simulink library "dspsrcs4"  (Simulink 6.0)
settings: Solver=ode45  SolverMode=SingleTasking  StartTime=0.0  StopTime=10.0  RelTol=1e-3
undefined symbols (not defined in the file or in its folder): dTypeID, Low
libraries: dspsigattribs x3, dspmtrx3 x2, dspswit3 x1
settings Model: RequirementInfo=9  CovMetricSettings=d  Creator=lelas  LastModifiedBy=sconahan  ExtModeAutoUpdateStatusClock=off
settings DataIOCC: SignalLoggingName=logsOut
settings OptimizationCC: BooleanDataType=off
settings DebuggingCC: CheckExecutionContextPreStartOutputMsg=on  CheckExecutionContextRuntimeOutputMsg=on  SolverPrmCheckMsg=none
settings HardwareCC: TargetUnknown=on
settings ModelReferenceCC: UpdateModelReferenceTargets=IfOutOfDate
settings SFSimCC: SFSimApplyToAllLibs=on  SFSimBuildMode=Incremental

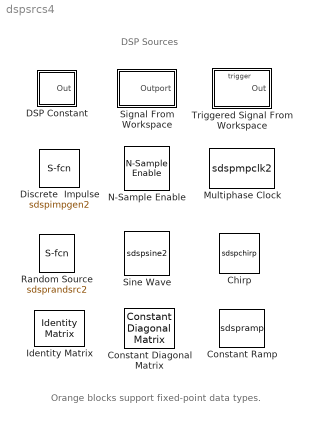
== system dspsrcs4 ==
  note: DSP Sources
  note: Orange blocks support fixed-point data types.
  Chirp : S-Function  FunctionName=sdspchirp  Parameters=sweep, mode, f0, f1, t1, Tsweep, phase, Ts, spf, beta, fmin,datatype  mask(Chirp){sweep=Linear, mode=Unidirectional, f0=1000, f1=4000, t1=1, Tsweep=1, phase=0, Ts=1/8000, spf=1, datatype=Double}
      mask prompts: sweep "Frequency sweep:"; mode "Sweep mode:"; f0 "Initial frequency (Hz):"; f1 "Target frequency (Hz):"; t1 "Target time (sec):"; Tsweep "Sweep time (sec):"; phase "Initial phase (radians):"; Ts "Sample time:"; spf "Samples per frame:"; datatype "Output data type:"
      mask help: Linear, Logarithmic, and Quadratic modes generate a swept-frequency cosine with instantaneous frequency values specified by the frequency and time parameters. The Swept cosine mode generates a swept-frequency cosine with a linear instantaneous output frequency that may differ from the one specified by the frequency and time parameters.
      mask init:
      | [t,y,txt] = dspblkchirp2('icon');
      | [beta,fmin] = dspblkchirp2('param',sweep, f0, f1, t1,Tsweep);
      mask Help: web(dspbhelp);
      mask StyleString: popup(Swept cosine|Linear|Logarithmic|Quadratic),popup(Unidirectional|Bidirectional),edit,edit,edit,edit,edit,edit,edit,popup(Double|Single)
      mask Display:
      | plot(t,y);
      | text(.2,.85,txt)
  Constant Diagonal Matrix : dspmtrx3/Constant Diagonal Matrix  q=ones(1,3)  frame=off  dataType=Inherit from 'Constant(s) along diagonal'  isSigned=on  wordLen=16  udDataType=sfix(16)  fracBitsMode=Best precision  numFracBits=15
  Constant Ramp : S-Function  FunctionName=sdspramp  Parameters=L, Slope, Offset,isCustomFloat,isSigned,dTypeID,wordLength,fracBits,fracBitsMode  mask(Constant Ramp){L=Rows, Slope=1, Offset=0, additionalParams=off, allowOverrides=on, dataType=Same as input, isSigned=on, wordLen=16, udDataType=sfix(16), fracBitsMode=Best precision, numFracBits=15}
      mask prompts: L "Ramp length equals number of:"; additionalParams "------- Show additional parameters --------"; allowOverrides "Allow overrides from DSP Fixed-Point Attributes blocks"; dataType "Output data type:"; isSigned "Signed"; wordLen "Word length:"; udDataType "User-defined data type (e.g. sfix(16), float('single')):"; fracBitsMode "Set fraction length in output to:"; numFracBits "Fraction length:"
      mask help:
      | Generate a ramp of length L, where L is either the number of rows or the number of columns of the input to the block.  Specify whether L is equal to the number of input rows or columns using the 'Ramp length equals number of' parameter.
      |
      | The output of this block is calculated using
      | output = [0:L-1] * slope + offset
      |
      | Note: Use the Ramp block in the Simulink Sources library to generate a ramp without providing block inputs.
      mask init:
      | x = [.1 .9];
      | if ~isa(Slope,'double')
      | 	s = 1;
      | else
      | 	s = Slope;
      | end
      | if (s >= 0), y =  s * [0 1];
      | else,   y =  s * [-1 0];  end;
      | [dtInfo,dTypeID]=dspblkramp('init');
      | isSigned=dtInfo.DataTypeIsSigned;
      | isCustomFloat=dtInfo.DataTypeIsCustomFloat;
      | wordLength=dtInfo.DataTypeWordLength;
      | fracBits=dtInfo.DataTypeFracOrMantBits;
      settings: CopyFcn=dspfixptcopycallback
      mask Help: web(dspbhelp);
      mask StyleString: popup(Rows|Columns),edit,edit,checkbox,checkbox,popup(Same as input|double|single|int8|uint8|int16|uint16|int32|uint32|boolean|Fixed-point|User-defined|Inherit via back propagation),checkbox,edit,edit,popup(Best precision|User-defined),edit
      mask CallbackString: |||||dspblkramp;|||dspblkramp;|dspblkramp;|
      mask TabNameString: Main,Main,Main,Main,Main,Data Types,Data Types,Data Types,Data Types,Data Types,Data Types
      mask Display: plot(x,y)
  DSP Constant : Subsystem  PropExecContextAcrossSSBoundary=on  mask(DSP Constant){Value=1, SampleMode=Discrete, discreteOutput=Sample-based, continuousOutput=Sample-based, sampTime=1, framePeriod=2, additionalParams=off, allowOverrides=on, dataType=Inherit from 'Constant value', isSigned=on, wordLen=16, udDataType=sfix(16), fracBitsMode=Best precision, numFracBits=15, InterpretAs1D=-inf, Ts=-inf, FramebasedOutput=-inf}
      mask prompts: Value "Constant value:"; SampleMode "Sample mode:"; discreteOutput "Output:"; continuousOutput "Output:"; sampTime "Sample time:"; framePeriod "Frame period:"; additionalParams "------- Show additional parameters --------"; allowOverrides "Allow overrides from DSP Fixed-Point Attributes blocks"; dataType "Output data type:"; isSigned "Signed"; wordLen "Word length:"; udDataType "User-defined data type:"; fracBitsMode "Set fraction length in output to:"; numFracBits "Fraction length:"; InterpretAs1D "old Interpret as 1D checkbox"; Ts "old Sample time/Frame period"; FramebasedOutput "old Frame-based output checkbox"
      mask help: Output a discrete-time or continuous-time constant.
      mask init:
      | dspblkdspconst2('init');
      | dspblkdspconst2('update');
      settings: CopyFcn=dspfixptcopycallback
      mask Help: web(dspbhelp);
      mask StyleString: edit,popup(Discrete|Continuous),popup(Sample-based (interpret vectors as 1-D)|Sample-based|Frame-based),popup(Sample-based (interpret vectors as 1-D)|Sample-based),edit,edit,checkbox,checkbox,popup(double|single|int8|uint8|int16|uint16|int32|uint32|boolean|Fixed-point|User-defined|Inherit from 'Constant value'|Inherit via back propagation),checkbox,edit,edit,popup(Best precision|User-defined),edit,edit,edit,edit
      mask CallbackString: |dspblkdspconst2;|dspblkdspconst2;|dspblkdspconst2;|||||dspblkdspconst2;|||dspblkdspconst2;|dspblkdspconst2;||||
      mask TabNameString: Main,Main,Main,Main,Main,Main,Main,Main,Data Types,Data Types,Data Types,Data Types,Data Types,Data Types,Main,Main,Main
      mask Display: disp(&1);
  Discrete  Impulse : S-Function  FunctionName=sdspimpgen2  Parameters=Delay, SampleTime,FrameSample,isCustomFloat,isSigned,dTypeID,wordLength,fracLength,[0 1]  mask(Discrete Impulse ){Delay=0, SampleTime=1, FrameSample=1, additionalParams=off, allowOverrides=on, dataType=double, isSigned=on, wordLen=16, udDataType=sfix(16), fracBitsMode=Best precision, numFracBits=15}
      mask prompts: Delay "Delay (samples):"; SampleTime "Sample time:"; FrameSample "Samples per frame:"; additionalParams "------- Show additional parameters --------"; allowOverrides "Allow overrides from DSP Fixed-Point Attributes blocks"; dataType "Output data type:"; isSigned "Signed"; wordLen "Word length:"; udDataType "User-defined data type (e.g. sfix(16), float('single')):"; fracBitsMode "Set fraction length in output to:"; numFracBits "Fraction length:"
      mask help: Output a discrete unit impulse. The impulse will be offset by the number of samples in the Delay parameter.
      mask init:
      | [x,y]=dspblkimpgen2('icon');
      | [dtInfo,dTypeID]=dspblkimpgen2('init');
      | isSigned=dtInfo.DataTypeIsSigned;
      | isCustomFloat=dtInfo.DataTypeIsCustomFloat;
      | wordLength=dtInfo.DataTypeWordLength;
      | fracLength=dtInfo.DataTypeFracOrMantBits;
      settings: CopyFcn=dspfixptcopycallback
      mask Help: web(dspbhelp);
      mask StyleString: edit,edit,edit,checkbox,checkbox,popup(double|single|int8|uint8|int16|uint16|int32|uint32|boolean|Fixed-point|User-defined|Inherit via back propagation),checkbox,edit,edit,popup(Best precision|User-defined),edit
      mask CallbackString: |||||dspblkimpgen2|||dspblkimpgen2|dspblkimpgen2|
      mask TabNameString: Main,Main,Main,Main,Main,Data Types,Data Types,Data Types,Data Types,Data Types,Data Types
      mask Display: plot(x,y)
  Identity Matrix : dspmtrx3/Identity Matrix  Inherit=off  N=5  Ts=1  dataType=double  isSigned=on  wordLen=16  udDataType=sfix(16)  fracBitsMode=Best precision  numFracBits=15
  Multiphase Clock : S-Function  FunctionName=sdspmpclk2  Parameters=ClkFreq, NumPhases, ActiveLevel, DutyCycle, StartPhase,DataType  mask(Multiphase Clock){ClkFreq=1, NumPhases=4, StartPhase=1, DutyCycle=3, ActiveLevel=High (1), DataType=Logical}
      mask prompts: ClkFreq "Clock frequency (Hz):"; NumPhases "Number of phases, N:"; StartPhase "Starting phase (1 to N):"; DutyCycle "Number of phase intervals over which clock is active (1 to N-1):"; ActiveLevel "Active level (polarity):"; DataType "Output data type"
      mask help: Generate a vector of N binary signals representing the N clock phases.
      mask init:
      | if isempty(NumPhases), s=&2;
      | else s=num2str(NumPhases);
      | end
      | s=[s '-Phase\nClock'];
      settings: CopyFcn=dspfixptcopycallback
      mask Help: web(dspbhelp);
      mask StyleString: edit,edit,edit,edit,popup(High (1)|Low (0)),popup(Logical|Boolean)
      mask Display: disp(s)
  N-Sample Enable : dspswit3/N-Sample Enable  N=8  ActiveLevel=Low (0)  reset=off  TriggerType=Rising edge  Ts=1  DataType=Logical
  Random Source : S-Function  FunctionName=sdsprandsrc2  Parameters=SrcType,NormMethod,double(CltLength),double(Min),double(Max),Mean,double(Var),RepMode,rawSeed,transformSeed,Inherit,SampMode,double(SampTime),SampFrame,DataType,OutComplex  mask(Random Source){SrcType=Uniform, NormMethod=Ziggurat, CltLength=12, Min=0, Max=1, Mean=0, Var=1, RepMode=Not repeatable, rawSeed=1, Inherit=off, SampMode=Discrete, SampTime=1, SampFrame=1, DataType=Double, OutComplex=Real}
      mask prompts: SrcType "Source type:"; NormMethod "Method:"; CltLength "Number of uniform values to sum:"; Min "Minimum:"; Max "Maximum:"; Var "Variance:"; RepMode "Repeatability:"; rawSeed "Initial seed:"; Inherit "Inherit output port attributes"; SampMode "Sample mode:"; SampTime "Sample time:"; SampFrame "Samples per frame:"; DataType "Output data type:"; OutComplex "Complexity:"
      mask help: Output a random signal with uniform or Gaussian (normal) distribution. Set output repeatability to Nonrepeatable (block randomly selects initial seed every time simulation starts), Repeatable (block randomly selects initial seed once and uses it every time simulation starts), or Specify seed (block uses specified initial seed every time simulation starts, producing repeatable output).
      mask init:
      | [x,y]=dspblkrandsrc2('icon');
      | if RepMode == 1
      | 	transformSeed=[];
      | else
      | 	transformSeed=eval(dspblkrandsrc2('seed'),'rawSeed');
      | end
      mask Help: web(dspbhelp);
      mask StyleString: popup(Uniform|Gaussian),popup(Ziggurat|Sum of uniform values),edit,edit,edit,edit,edit,popup(Specify seed|Repeatable|Not repeatable),edit,checkbox,popup(Discrete|Continuous),edit,edit,popup(Double|Single),popup(Real|Complex)
      mask CallbackString:
      | dspblkrandsrc2;|dspblkrandsrc2;
      | ||||||dspblkrandsrc2;||dspblkrandsrc2;|dspblkrandsrc2;||||
      mask Display: plot(x,y);
  Signal From Workspace : Subsystem  PropExecContextAcrossSSBoundary=on  mask(Signal From Workspace){X=1:10, Ts=1, nsamps=1, OutputAfterFinalValue=Setting to zero}
      mask prompts: X "Signal:"; Ts "Sample time:"; nsamps "Samples per frame:"; OutputAfterFinalValue "Form output after final data value by:"
      mask help:
      | Output signal samples obtained from the MATLAB workspace at successive sample times.  A signal matrix is interpreted as having one channel per column.  Signal columns may be buffered into frames by specifying a number of samples per frame greater than 1.
      |
      | An M x N x P signal array outputs M x N matrices at successive sample times.  The samples per frame must be equal to 1 for 3 dimensional signal arrays.
      mask init:
      | [s,Ts] = dspblksfw2('init', X,Ts,nsamps);
      settings: CopyFcn=dspfixptcopycallback
      mask Help: web(dspbhelp);
      mask StyleString: edit,edit,edit,popup(Setting to zero|Holding final value|Cyclic repetition)
      mask Display: disp(&1)
  Sine Wave : S-Function  FunctionName=sdspsine2  Parameters=Amplitude,Frequency,Phase,SampleMode,OutComplex,CompMethod,SampleTime,SamplesPerFrame,ResetState,TableSize,isCustomFloat,isSigned,dTypeID,wordLength,fracBits  mask(Sine Wave){Amplitude=1, Frequency=100, Phase=0, SampleMode=Discrete, OutComplex=Real, CompMethod=Trigonometric fcn, TableSize=Speed, SampleTime=1/1000, SamplesPerFrame=1, additionalParams=off, allowOverrides=on, dataType=double, wordLen=16, udDataType=sfix(16), fracBitsMode=Best precision, numFracBits=15, ResetState=Restart at time zero}
      mask prompts: Frequency "Frequency (Hz):"; Phase "Phase offset (rad):"; SampleMode "Sample mode:"; OutComplex "Output complexity:"; CompMethod "Computation method:"; TableSize "Optimize table for:"; SampleTime "Sample time:"; SamplesPerFrame "Samples per frame:"; additionalParams "------- Show additional parameters --------"; allowOverrides "Allow overrides from DSP Fixed-Point Attributes blocks"; dataType "Output data type:"; wordLen "Word length:"; udDataType "User-defined data type (e.g. sfix(16), float('single')):"; fracBitsMode "Set fraction length in output to:"; numFracBits "Fraction length:"; ResetState "Resetting states when re-enabled:"
      mask help: Output samples of a sinusoid. To generate more than one sinusoid simultaneously, enter a vector of values for the Amplitude, Frequency, and Phase offset parameters.
      mask init:
      | [x,y] = dspblksine('icon');
      | [dtInfo,dTypeID]=dspblksine('init');
      | isSigned=dtInfo.DataTypeIsSigned;
      | isCustomFloat=dtInfo.DataTypeIsCustomFloat;
      | wordLength=dtInfo.DataTypeWordLength;
      | fracBits=dtInfo.DataTypeFracOrMantBits;
      | dType=dataType;
      settings: CopyFcn=dspfixptcopycallback
      mask Help: web(dspbhelp);
      mask StyleString: edit,edit,edit,popup(Discrete|Continuous),popup(Real|Complex),popup(Trigonometric fcn|Table lookup|Differential),popup(Speed|Memory),edit,edit,checkbox,checkbox,popup(double|single|Fixed-point|User-defined|Inherit via back propagation),edit,edit,popup(Best precision|User-defined),edit,popup(Restart at time zero|Catch up to simulation time)
      mask CallbackString: |||dspblksine;||dspblksine;||||||dspblksine||dspblksine|dspblksine||
      mask TabNameString: Main,Main,Main,Main,Main,Main,Main,Main,Main,Main,Main,Data Types,Data Types,Data Types,Data Types,Data Types,Main
      mask Display:
      | plot(x,y)
      | text(3.25,.75,'DSP');
  Triggered Signal From Workspace : Subsystem  TreatAsAtomicUnit=on  PropExecContextAcrossSSBoundary=on  mask(Triggered Signal From Workspace){Signal=1:10, TriggerType=Falling edge, ic=0, SamplesPerFrame=1, OutputAfterFinalValue=Setting to zero}
      mask prompts: TriggerType "Trigger type:"; ic "Initial output:"; SamplesPerFrame "Samples per frame:"; OutputAfterFinalValue "Form output after final data value by:"
      mask help: Output successive signal samples obtained from the MATLAB workspace when a trigger event occurs. A signal matrix is interpreted as having one channel per column. Signal columns may be buffered into frames by specifying a number of samples per frame greater than 1. An M x N x P signal array outputs M x N matrices when a trigger event occurs. The samples per frame must be equal to 1 for 3 dimensional signal arrays.
      mask init:
      | s = dspblktsfw2('init', Signal,SamplesPerFrame);
      settings: CopyFcn=dspfixptcopycallback
      mask Help: web(dspbhelp);
      mask StyleString: edit,popup(Rising edge|Falling edge|Either edge),edit,edit,popup(Setting to zero|Holding final value|Cyclic repetition)
      mask Display: disp(&1);

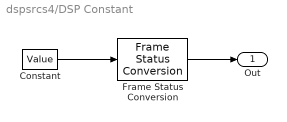
== system dspsrcs4/DSP Constant ==
  Constant : Constant  Value=Value  VectorParams1D=off  SampleTime=sampTime
  Frame Status Conversion : dspsigattribs/Frame Status Conversion  growRefPort=off  outframe=Sample-based
  Out : Outport
  wires:
  Frame Status Conversion/1 -> Out/1
  Constant/1 -> Frame Status Conversion/1

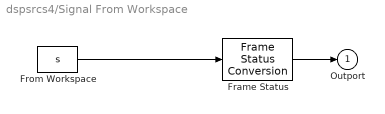
== system dspsrcs4/Signal From Workspace ==
  Frame Status : dspsigattribs/Frame Status Conversion  growRefPort=off  outframe=Sample-based
  From Workspace : FromWorkspace  VariableName=s  SampleTime=Ts  Interpolate=off  OutputAfterFinalValue=Setting to zero
  Outport : Outport  InitialOutput=0
  wires:
  From Workspace/1 -> Frame Status/1
  Frame Status/1 -> Outport/1

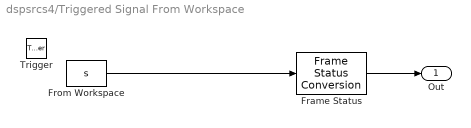
== system dspsrcs4/Triggered Signal From Workspace ==
  Trigger : TriggerPort  TriggerType=falling  StatesWhenEnabling=reset  ZeroCross=off
  Frame Status : dspsigattribs/Frame Status Conversion  growRefPort=off  outframe=Sample-based
  From Workspace : FromWorkspace  VariableName=s  Interpolate=off  OutputAfterFinalValue=Setting to zero
  Out : Outport  InitialOutput=ic
  wires:
  Frame Status/1 -> Out/1
  From Workspace/1 -> Frame Status/1
